simulink subsystem "attComputer"  (R2021a)
settings: Solver=VariableStepAuto  StartTime=0.0  StopTime=10.0  RelTol=1e-3
libraries: attitude_library x2
settings Model: Creator=Laura  LastModifiedBy=Laura

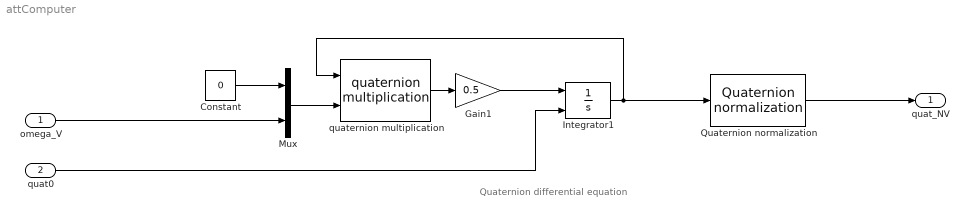
== system attComputer ==
  note: Quaternion differential equation
  omega_V : Inport
  quat0 : Inport  Port=2
  Constant : Constant  Value=0
  Gain1 : Gain  Gain=0.5
  Integrator1 : Integrator  InitialConditionSource=external  InitialCondition=[1;0;0;0]
  Mux : Mux  Inputs=2
  Quaternion normalization : attitude_library/Quaternion normalization  SystemSampleTime=-1  VariantActivationTime=update diagram  Latency=0  AutoFrameSizeCalculation=off
      settings: SourceProductName=Attitude library
  quaternion multiplication : attitude_library/quaternion multiplication  SystemSampleTime=-1  VariantActivationTime=update diagram  Latency=0  AutoFrameSizeCalculation=off
      settings: SourceProductName=Attitude library
  quat_NV : Outport
  wires:
  Gain1/1 -> Integrator1/1
  Mux/1 -> quaternion multiplication/2
  Constant/1 -> Mux/1
  quaternion multiplication/1 -> Gain1/1
  Integrator1/1 -> quaternion multiplication/1, Quaternion normalization/1
  omega_V/1 -> Mux/2
  Quaternion normalization/1 -> quat_NV/1
  quat0/1 -> Integrator1/2
